simulink model "SYHW_Zscan"  (Simulink 8.1)
settings: Solver=ode5  SolverMode=SingleTasking  StartTime=0.0  StopTime=inf  FixedStep=Ts  RelTol=1e-3
PreLoadFcn:
  | Ts=20e-6;Ts_eHS=8e-7;parameters3;
PostLoadFcn:
  | Ts=20e-6;Ts_eHS=8e-7;parameters3;
InitFcn:
  | Ts=20e-6;Ts_eHS=8e-7;parameters3;
StartFcn:
  | Ts=20e-6;Ts_eHS=8e-7;parameters3;
undefined symbols (not defined in the file or in its folder): Fnom, opsimget, p, SW01
undefined symbols (not defined in the file): LmSI, LrSI, LsSI, RrSI, RsSI
libraries: rtlab x35, rtio_opalrt_common x13, efs_cpuhilios_crtl_lib x4, cpuhilios_lib x4, simulink x3, dspsigops x3, powerlib_extras x1, powerlib_meascontrol x1, rteventslib x1, cpuconverter_lib x1
(part 2 of 2)

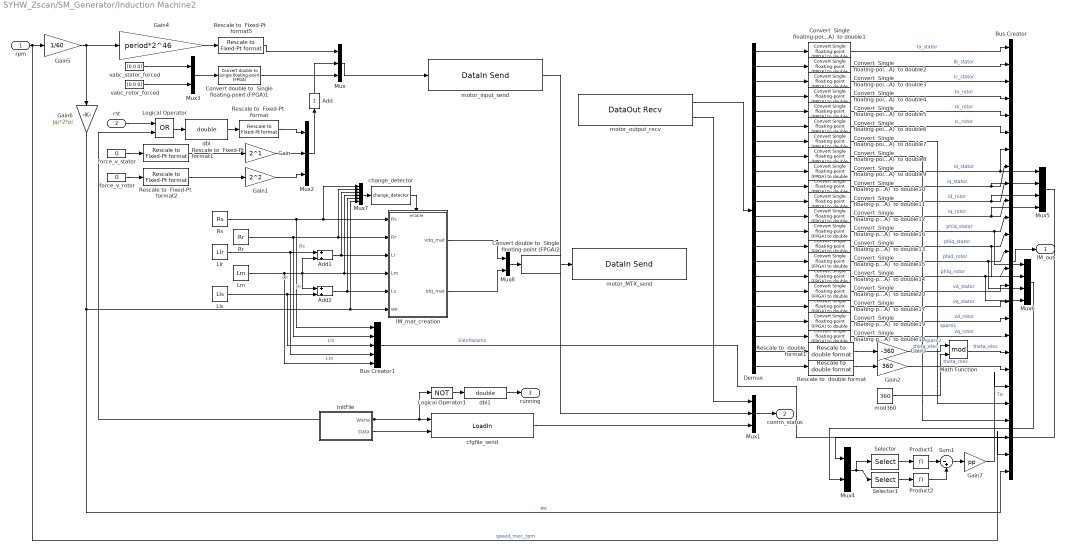
== system SYHW_Zscan/SM_Generator/Induction Machine2 ==
  rpm : Inport  PortDimensions=1
  rst : Inport  Port=2
  Add : Sum  Inputs=+
  Add1 : Sum
  Add2 : Sum
  Bus Creator : BusCreator  Inputs=26
  Bus Creator1 : BusCreator  Inputs=5
  Convert  Single floating-point (FPGA)  to double{1..20} (20 alike) : rtlab/Miscellaneous/Convert  Single floating-point (FPGA)  to double
  Convert double to  Single floating-point (FPGA)1 : rtlab/Miscellaneous/Convert double to  Single floating-point (FPGA)
  Convert double to  Single floating-point (FPGA)2 : rtlab/Miscellaneous/Convert double to  Single floating-point (FPGA)
  Demux : Demux  Outputs=22
  Gain : Gain  Gain=2^1  OutDataTypeStr=uint32
  Gain1 : Gain  Gain=2^2  OutDataTypeStr=uint32
  Gain2 : Gain  Gain=360
  Gain3 : Gain  Gain=-360
  Gain4 : Gain  Gain=period*2^46
  Gain5 : Gain  Gain=1/60
  Gain6 : Gain  Gain=pp*2*pi
  Gain7 : Gain  Gain=pp
  IM_mat_creation : Subsystem
  InitFile : Subsystem
      mask Display:
      | patch([0 0.5 0.7 0],[1 1 0 0],[0.7 0.75 0.9]);
      | patch([1 0.53 0.73 1],[1 1 0 0],[1 0.8 0.7]);
      | port_label('output',2,'Data');
      | 
      | port_label('output',1,'En');
  Llr : Constant  Value=Llr
  Lls : Constant  Value=Lls
  Lm : Constant  Value=Lm
  Logical Operator : Logic  Operator=OR  AllPortsSameDT=off  OutDataTypeStr=boolean
  Logical Operator1 : Logic  Operator=NOT  AllPortsSameDT=off  OutDataTypeStr=boolean
  Math Function : Math  Operator=mod  SaturateOnIntegerOverflow=on
  Mux : Mux  Inputs=3
  Mux1 : Mux  Inputs=3
  Mux2 : Mux  Inputs=3
  Mux3 : Mux  Inputs=2
  Mux4 : Mux  Inputs=2
  Mux5 : Mux
  Mux6 : Mux
  Mux7 : Mux  Inputs=6
  Mux8 : Mux  Inputs=2
  Product1 : Product  Inputs=1  SaturateOnIntegerOverflow=on  InputSameDT=on  OutDataTypeStr=Inherit: Same as first input
  Product2 : Product  Inputs=1  SaturateOnIntegerOverflow=on  InputSameDT=on  OutDataTypeStr=Inherit: Same as first input
  Rescale to  Fixed-Pt  format : rtlab/Miscellaneous/Rescale to  Fixed-Pt  format  FormatType=Unsigned  N=1  Q=0
  Rescale to  Fixed-Pt  format1 : rtlab/Miscellaneous/Rescale to  Fixed-Pt  format  FormatType=Unsigned  N=6  Q=0
  Rescale to  Fixed-Pt  format2 : rtlab/Miscellaneous/Rescale to  Fixed-Pt  format  FormatType=Unsigned  N=1  Q=0
  Rescale to  Fixed-Pt  format5 : rtlab/Miscellaneous/Rescale to  Fixed-Pt  format  FormatType=Signed (2's complement)  N=32  Q=0
  Rescale to  double format : rtlab/Miscellaneous/Rescale to  double format  FormatType=Unsigned  N=32  Q=32
  Rescale to  double format1 : rtlab/Miscellaneous/Rescale to  double format  FormatType=Unsigned  N=32  Q=32
  Rr : Constant  Value=Rr
  Rs : Constant  Value=Rs
  Selector : Selector  InputPortWidth=8  IndexOptions=Index vector (dialog)  Indices=[1 6]  OutputSizes=1
  Selector1 : Selector  InputPortWidth=8  IndexOptions=Index vector (dialog)  Indices=[2 5]  OutputSizes=1
  Sum1 : Sum  Inputs=|-+  SaturateOnIntegerOverflow=on  InputSameDT=on  OutDataTypeStr=Inherit: Same as first input
  cfgfile_send : rtio_opalrt_common/LoadIn  CtrlName='eHS Ctrl'  FcnNos=27  width=10  portType=uint32
      settings: AttributesFormatString=%<CtrlName>
  change_detector : cpuhilios_lib/Aout_Mapping&Adjustments/change_detector
  dbl : DataTypeConversion  OutDataTypeStr=double
  dbl1 : DataTypeConversion  OutDataTypeStr=double
  force_v_rotor : Constant  Value=0
  force_v_stator : Constant  Value=0
  mod360 : Constant  Value=360
  motor_MTX_send : rtio_opalrt_common/DataIn Send  CtrlName='eHS Ctrl'  FcnNos=23  width=32  portType=uint32  checkVersion=off  expectedId=0  expectedVersion=0  opComp=>=
      settings: AttributesFormatString=%<CtrlName>
  motor_input_send : rtio_opalrt_common/DataIn Send  CtrlName='eHS Ctrl'  FcnNos=22  width=8  portType=uint32  checkVersion=off  expectedId=0  expectedVersion=0  opComp=>=
      settings: AttributesFormatString=%<CtrlName>
  motor_output_recv : rtio_opalrt_common/DataOut Recv  CtrlName='eHS Ctrl'  FcnNos=3  width=22  portType=uint32  sampleTime=0  checkVersion=off  expectedId=0  expectedVersion=0  opComp=>=
      settings: AttributesFormatString=%<CtrlName>
  vabc_rotor_forced : Constant  Value=[0 0 0]
  vabc_stator_forced : Constant  Value=[0 0 0]
  IM_out : Outport
  comm_status : Outport  Port=2
  running : Outport  Port=3
  wires:
  Bus Creator1/1 -> Bus Creator/24  "ElecParams"
  Gain5/1 -> Gain4/1, Gain6/1
  dbl1/1 -> running/1
  Logical Operator1/1 -> dbl1/1
  dbl/1 -> Rescale to  Fixed-Pt  format/1
  Rescale to  Fixed-Pt  format/1 -> Mux2/1
  Logical Operator/1 -> dbl/1
  Demux/1 -> Convert  Single floating-point (FPGA)  to double1/1
  rpm/1 -> Bus Creator/25, Gain5/1  "speed_mec_rpm"
  Gain1/1 -> Mux2/3
  Rescale to  Fixed-Pt  format2/1 -> Gain1/1
  force_v_rotor/1 -> Rescale to  Fixed-Pt  format2/1
  Gain/1 -> Mux2/2
  force_v_stator/1 -> Rescale to  Fixed-Pt  format1/1
  Mux2/1 -> Add/1
  Rescale to  Fixed-Pt  format1/1 -> Gain/1
  rst/1 -> Logical Operator/1
  motor_output_recv/1 -> Demux/1
  InitFile/1(Wena) -> Logical Operator1/1, cfgfile_send/1, Logical Operator/2
  Mux/1 -> motor_input_send/1
  Gain4/1 -> Rescale to  Fixed-Pt  format5/1
  Convert double to  Single floating-point (FPGA)1/1 -> Mux/3
  motor_input_send/1 -> Mux1/2
  motor_output_recv/2 -> Mux1/1
  vabc_stator_forced/1 -> Mux3/1
  cfgfile_send/1 -> Mux1/3
  Mux1/1 -> comm_status/1
  InitFile/2(Data) -> cfgfile_send/2
  Rescale to  Fixed-Pt  format5/1 -> Mux/1
  Add/1 -> Mux/2
  Convert  Single floating-point (FPGA)  to double1/1 -> Bus Creator/1  "Ia_stator"
  Rescale to  double format/1 -> Gain2/1
  Rescale to  double format1/1 -> Gain3/1
  Gain2/1 -> Bus Creator/20  "theta_mec"
  Gain3/1 -> Math Function/1  "theta_elec"
  Mux3/1 -> Convert double to  Single floating-point (FPGA)1/1
  vabc_rotor_forced/1 -> Mux3/2
  Convert  Single floating-point (FPGA)  to double2/1 -> Bus Creator/2  "Ib_stator"
  Demux/2 -> Convert  Single floating-point (FPGA)  to double2/1
  Demux/3 -> Convert  Single floating-point (FPGA)  to double3/1
  Convert  Single floating-point (FPGA)  to double3/1 -> Bus Creator/3  "Ic_stator"
  Convert  Single floating-point (FPGA)  to double4/1 -> Bus Creator/4  "Ia_rotor"
  Demux/4 -> Convert  Single floating-point (FPGA)  to double4/1
  Convert  Single floating-point (FPGA)  to double5/1 -> Bus Creator/5  "Ib_rotor"
  Demux/5 -> Convert  Single floating-point (FPGA)  to double5/1
  Convert  Single floating-point (FPGA)  to double6/1 -> Bus Creator/6  "Ic_rotor"
  Demux/6 -> Convert  Single floating-point (FPGA)  to double6/1
  Convert  Single floating-point (FPGA)  to double7/1 -> Bus Creator/22  "spare1"
  Demux/7 -> Convert  Single floating-point (FPGA)  to double7/1
  Convert  Single floating-point (FPGA)  to double8/1 -> Bus Creator/23  "spare2"
  Demux/8 -> Convert  Single floating-point (FPGA)  to double8/1
  Convert  Single floating-point (FPGA)  to double9/1 -> Bus Creator/7, Mux5/1  "id_stator"
  Demux/9 -> Convert  Single floating-point (FPGA)  to double9/1
  Convert  Single floating-point (FPGA)  to double10/1 -> Bus Creator/8, Mux5/2  "iq_stator"
  Demux/10 -> Convert  Single floating-point (FPGA)  to double10/1
  Convert  Single floating-point (FPGA)  to double11/1 -> Bus Creator/9, Mux5/3  "id_rotor"
  Demux/11 -> Convert  Single floating-point (FPGA)  to double11/1
  Convert  Single floating-point (FPGA)  to double12/1 -> Bus Creator/10, Mux5/4  "iq_rotor"
  Demux/12 -> Convert  Single floating-point (FPGA)  to double12/1
  Convert  Single floating-point (FPGA)  to double16/1 -> Bus Creator/11, Mux6/1  "phid_stator"
  Demux/13 -> Convert  Single floating-point (FPGA)  to double16/1
  Convert  Single floating-point (FPGA)  to double13/1 -> Bus Creator/12, Mux6/2  "phiq_stator"
  Demux/14 -> Convert  Single floating-point (FPGA)  to double13/1
  Convert  Single floating-point (FPGA)  to double15/1 -> Bus Creator/13, Mux6/3  "phid_rotor"
  Demux/15 -> Convert  Single floating-point (FPGA)  to double15/1
  Convert  Single floating-point (FPGA)  to double14/1 -> Bus Creator/14, Mux6/4  "phiq_rotor"
  Demux/16 -> Convert  Single floating-point (FPGA)  to double14/1
  Convert  Single floating-point (FPGA)  to double20/1 -> Bus Creator/15  "vd_stator"
  Convert  Single floating-point (FPGA)  to double17/1 -> Bus Creator/16  "vq_stator"
  Convert  Single floating-point (FPGA)  to double19/1 -> Bus Creator/17  "vd_rotor"
  Convert  Single floating-point (FPGA)  to double18/1 -> Bus Creator/18  "vq_rotor"
  Demux/17 -> Convert  Single floating-point (FPGA)  to double20/1
  Demux/18 -> Convert  Single floating-point (FPGA)  to double17/1
  Demux/19 -> Convert  Single floating-point (FPGA)  to double19/1
  Demux/20 -> Convert  Single floating-point (FPGA)  to double18/1
  Demux/21 -> Rescale to  double format1/1
  Demux/22 -> Rescale to  double format/1
  Bus Creator/1 -> IM_out/1
  Mux8/1 -> Convert double to  Single floating-point (FPGA)2/1
  Rs/1 -> Bus Creator1/1, IM_mat_creation/1(Rs), Mux7/1  "Rs"
  Rr/1 -> Bus Creator1/2, IM_mat_creation/2(Rr), Mux7/2  "Rr"
  Llr/1 -> Bus Creator1/4, Add1/1  "Llr"
  Lm/1 -> Bus Creator1/5, IM_mat_creation/4(Lm), Mux7/4, Add2/1, Add1/2  "Lm"
  Lls/1 -> Bus Creator1/3, Add2/2  "Lls"
  IM_mat_creation/1(vdq_mat) -> Mux8/1
  IM_mat_creation/2(idq_mat) -> Mux8/2
  Gain6/1 -> Bus Creator/26, IM_mat_creation/6(we), Mux7/6  "we"
  Selector/1 -> Product1/1
  Selector1/1 -> Product2/1
  Product2/1 -> Sum1/2
  Product1/1 -> Sum1/1
  Sum1/1 -> Gain7/1
  Mux4/1 -> Selector1/1, Selector/1
  Gain7/1 -> Bus Creator/21  "Te"
  Mux5/1 -> Mux4/1
  Mux6/1 -> Mux4/2
  Add1/1 -> IM_mat_creation/3(Lr), Mux7/3
  Add2/1 -> IM_mat_creation/5(Ls), Mux7/5
  Convert double to  Single floating-point (FPGA)2/1 -> motor_MTX_send/1
  Mux7/1 -> change_detector/1
  change_detector/1 -> IM_mat_creation/Enable
  Math Function/1 -> Bus Creator/19  "theta_elec"
  mod360/1 -> Math Function/2

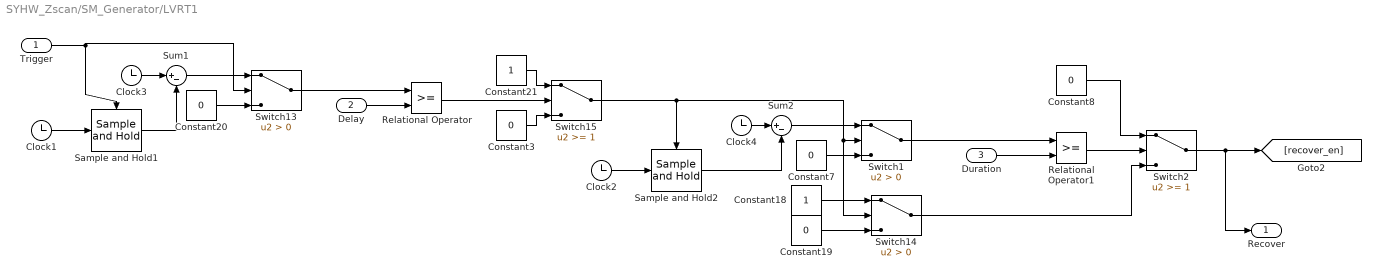
== system SYHW_Zscan/SM_Generator/LVRT1 ==
  Trigger : Inport
  Delay : Inport  Port=2
  Duration : Inport  Port=3
  Clock{1..4} (4 alike) : Clock
      Clock3 settings: DisableCoverage=on
      Clock4 settings: DisableCoverage=on
  Constant18 : Constant
  Constant{3,7..8,19..20} (5 alike) : Constant  Value=0
  Constant21 : Constant
  Relational Operator : RelationalOperator  OutDataTypeStr=boolean
  Relational Operator1 : RelationalOperator  OutDataTypeStr=boolean
  Sample and Hold1 : dspsigops/Sample and Hold  trig=Rising edge  initCond=0  latchinput=off
  Sample and Hold2 : dspsigops/Sample and Hold  trig=Rising edge  initCond=0  latchinput=off
  Sum1 : Sum  DisableCoverage=on  Inputs=|+-  SaturateOnIntegerOverflow=on  InputSameDT=on  OutDataTypeStr=Inherit: Same as first input
  Sum2 : Sum  DisableCoverage=on  Inputs=|+-  SaturateOnIntegerOverflow=on  InputSameDT=on  OutDataTypeStr=Inherit: Same as first input
  Switch1 : Switch  Criteria=u2 > Threshold
  Switch13 : Switch  Criteria=u2 > Threshold
  Switch14 : Switch  Criteria=u2 > Threshold
  Switch15 : Switch  Threshold=1
  Switch2 : Switch  Threshold=1
  Recover : Outport
  wires:
  Duration/1 -> Relational Operator1/2
  Switch1/1 -> Relational Operator1/1
  Relational Operator1/1 -> Switch2/2
  Relational Operator/1 -> Switch15/2
  Delay/1 -> Relational Operator/2
  Switch13/1 -> Relational Operator/1
  Clock2/1 -> Sample and Hold2/1
  Sum2/1 -> Switch1/1
  Constant18/1 -> Switch14/1
  Sample and Hold2/1 -> Sum2/2
  Constant8/1 -> Switch2/1
  Clock4/1 -> Sum2/1
  Constant7/1 -> Switch1/3
  Switch14/1 -> Switch2/3
  Constant19/1 -> Switch14/3
  Sample and Hold1/1 -> Sum1/2
  Clock1/1 -> Sample and Hold1/1
  Constant20/1 -> Switch13/3
  Sum1/1 -> Switch13/1
  Constant21/1 -> Switch15/1
  Constant3/1 -> Switch15/3
  Clock3/1 -> Sum1/1
  Switch15/1 -> Sample and Hold2/Trigger, Switch14/2, Switch1/2
  Trigger/1 -> Switch13/2, Sample and Hold1/Trigger
  Switch2/1 -> Recover/1, [recover_en]

== system SYHW_Zscan/SM_Generator/Motor voltage ==
  Uscan_abc : Inport
  Ugrid_abc : Inport  Port=2
  Add4 : Sum
  Add8 : Sum
  Add9 : Sum
  Bus Creator : BusCreator  Inputs=3
  Demux : Demux  Outputs=3
  Demux1 : Demux  Outputs=3
  Gain1 : Gain  Gain=sqrt(2/3)
  Product : Product  RndMeth=Zero
  Uabc : Sin  Frequency=100*pi  Phase=[0 -2/3*pi 2/3*pi]  SampleTime=0
  Out1 : Outport
  wires:
  Ugrid_abc/1 -> Gain1/1
  Uabc/1 -> Product/1
  Gain1/1 -> Product/2
  Add4/1 -> Bus Creator/1  "Ua_total"
  Add9/1 -> Bus Creator/3  "Uc_total"
  Add8/1 -> Bus Creator/2  "Ub_total"
  Product/1 -> Demux/1
  Demux1/3 -> Add9/2
  Demux1/2 -> Add8/2
  Demux1/1 -> Add4/2
  Uscan_abc/1 -> Demux1/1
  Demux/1 -> Add4/1
  Demux/2 -> Add8/1
  Demux/3 -> Add9/1
  Bus Creator/1 -> Out1/1

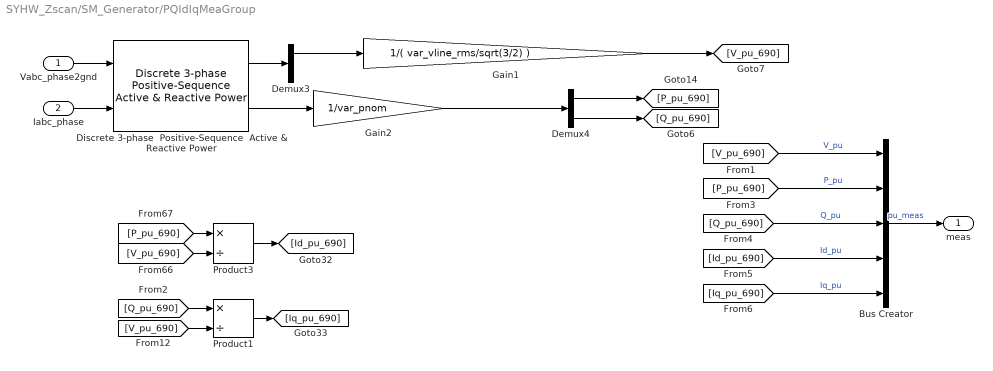
== system SYHW_Zscan/SM_Generator/PQIdIqMeaGroup ==
  Vabc_phase2gnd : Inport
  Iabc_phase : Inport  Port=2
  Bus Creator : BusCreator  Inputs=5
  Demux3 : Demux  Outputs=2
  Demux4 : Demux  Outputs=2
  Discrete 3-phase  Positive-Sequence  Active & Reactive Power : powerlib_extras/Discrete Measurements/Discrete 3-phase  Positive-Sequence  Active & Reactive Power  Freq=50  Par_Vinit=[0 0]  Par_Iinit=[0 0]  Ts=Ts
  Gain1 : Gain  Gain=1/( var_vline_rms/sqrt(3/2) )
  Gain2 : Gain  Gain=1/var_pnom
  Product1 : Product  Inputs=*/  RndMeth=Zero
  Product3 : Product  Inputs=*/  RndMeth=Zero
  meas : Outport
  wires:
  Iabc_phase/1 -> Discrete 3-phase  Positive-Sequence  Active & Reactive Power/2
  Vabc_phase2gnd/1 -> Discrete 3-phase  Positive-Sequence  Active & Reactive Power/1
  Discrete 3-phase  Positive-Sequence  Active & Reactive Power/1 -> Demux3/1
  Demux3/1 -> Gain1/1
  Discrete 3-phase  Positive-Sequence  Active & Reactive Power/2 -> Gain2/1
  Demux4/1 -> [P_pu_690]
  Demux4/2 -> [Q_pu_690]
  Product1/1 -> [Iq_pu_690]
  [Q_pu_690] -> Product1/1
  [V_pu_690] -> Product1/2
  [P_pu_690] -> Product3/1
  Product3/1 -> [Id_pu_690]
  [V_pu_690] -> Product3/2
  [P_pu_690] -> Bus Creator/2  "P_pu"
  [V_pu_690] -> Bus Creator/1  "V_pu"
  [Q_pu_690] -> Bus Creator/3  "Q_pu"
  [Iq_pu_690] -> Bus Creator/5  "Iq_pu"
  [Id_pu_690] -> Bus Creator/4  "Id_pu"
  Bus Creator/1 -> meas/1  "pu_meas"
  Gain1/1 -> [V_pu_690]
  Gain2/1 -> Demux4/1

== system SYHW_Zscan/SM_Generator/QuadEncoders ==
  Slot1B_1 : Inport
  Power base for the Generator3 : Gain  Gain=60*Fnom/p  SaturateOnIntegerOverflow=on  OutDataTypeStr=Inherit: Same as input  ParamDataTypeStr=Inherit: Same as input
  Scope : Scope
      settings: SaveName=ScopeData7
  Speed scaling : Subsystem
  To_FPGA : Outport
  wires:
  Slot1B_1/1 -> Power base for the Generator3/1
  Speed scaling/1(DataIN) -> To_FPGA/1
  Power base for the Generator3/1 -> Scope/1, Speed scaling/2(QuadEnc2), Speed scaling/1(QuadEnc1)

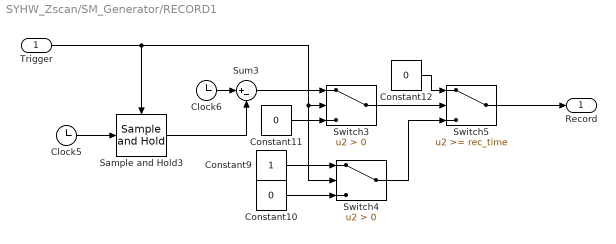
== system SYHW_Zscan/SM_Generator/RECORD1 ==
  Trigger : Inport
  Clock5 : Clock
  Clock6 : Clock
      settings: DisableCoverage=on
  Constant10 : Constant  Value=0
  Constant11 : Constant  Value=0
  Constant12 : Constant  Value=0
  Constant9 : Constant
  Sample and Hold3 : dspsigops/Sample and Hold  trig=Rising edge  initCond=0  latchinput=off
  Sum3 : Sum  DisableCoverage=on  Inputs=|+-  SaturateOnIntegerOverflow=on  InputSameDT=on  OutDataTypeStr=Inherit: Same as first input
  Switch3 : Switch  Criteria=u2 > Threshold
  Switch4 : Switch  Criteria=u2 > Threshold
  Switch5 : Switch  Threshold=rec_time
  Record : Outport
  wires:
  Constant10/1 -> Switch4/3
  Constant12/1 -> Switch5/1
  Sample and Hold3/1 -> Sum3/2
  Clock6/1 -> Sum3/1
  Switch4/1 -> Switch5/3
  Constant11/1 -> Switch3/3
  Constant9/1 -> Switch4/1
  Sum3/1 -> Switch3/1
  Clock5/1 -> Sample and Hold3/1
  Switch3/1 -> Switch5/2
  Trigger/1 -> Switch4/2, Switch3/2, Sample and Hold3/Trigger
  Switch5/1 -> Record/1

== system SYHW_Zscan/SM_Generator/pp2pg ==
  Vabc_pp : Inport
  Add : Sum  Inputs=+-
  Add1 : Sum  Inputs=-+
  Add2 : Sum  Inputs=-+
  Demux : Demux  Outputs=3
  Gain2 : Gain  Gain=1/3
  Mux12 : Mux  Inputs=3
  Vabc : Outport
  wires:
  Mux12/1 -> Gain2/1
  Demux/1 -> Add/1, Add1/1
  Demux/3 -> Add/2, Add2/2
  Add/1 -> Mux12/1
  Gain2/1 -> Vabc/1
  Demux/2 -> Add1/2, Add2/1
  Add1/1 -> Mux12/2
  Add2/1 -> Mux12/3
  Vabc_pp/1 -> Demux/1

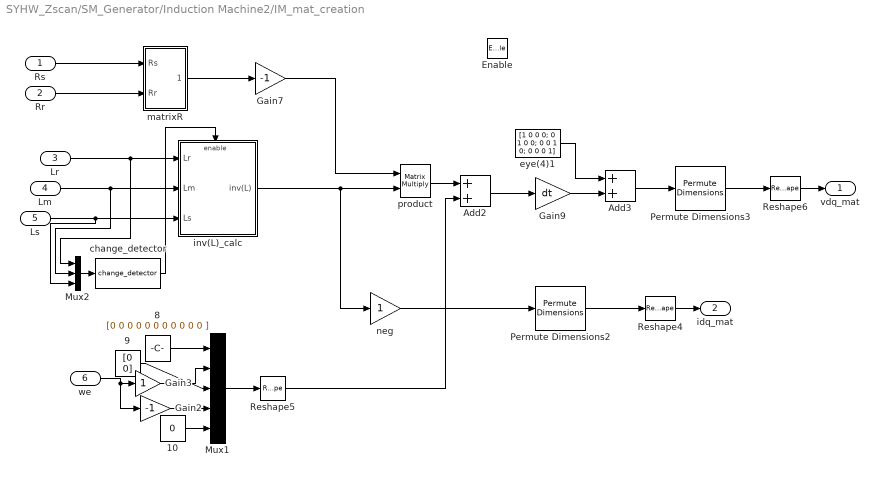
== system SYHW_Zscan/SM_Generator/Induction Machine2/IM_mat_creation ==
  Rs : Inport
  Rr : Inport  Port=2
  Lr : Inport  Port=3
  Lm : Inport  Port=4
  Ls : Inport  Port=5
  we : Inport  Port=6
  Enable : EnablePort
  10 : Constant  Value=0
  8 : Constant  Value=[0 0 0 0 0 0 0 0 0 0 0 ]
  9 : Constant  Value=[0 0]
  Add2 : Sum
  Add3 : Sum
  Gain2 : Gain  Gain=-1
  Gain3 : Gain
  Gain7 : Gain  Gain=-1
  Gain9 : Gain  Gain=dt
  Mux1 : Mux  Inputs=[11 1 2 1 1]
  Mux2 : Mux  Inputs=3
  Permute Dimensions2 : PermuteDimensions
  Permute Dimensions3 : PermuteDimensions
  Reshape4 : Reshape
  Reshape5 : Reshape  OutputDimensionality=Customize  OutputDimensions=[4,4]
  Reshape6 : Reshape
  change_detector : cpuhilios_lib/Aout_Mapping&Adjustments/change_detector
  eye(4)1 : Constant  Value="[1 0 0 0; 0 1 0 0; 0 0  1  0;  0  0  0  1]"
  inv(L)_calc : Subsystem
  matrixR : Subsystem
  neg : Gain
  product : Product  Multiplication=Matrix(*)
  vdq_mat : Outport
  idq_mat : Outport  Port=2
  wires:
  Gain3/1 -> Mux1/2
  10/1 -> Mux1/5
  9/1 -> Mux1/3
  Gain2/1 -> Mux1/4
  we/1 -> Gain2/1, Gain3/1
  8/1 -> Mux1/1
  Mux1/1 -> Reshape5/1
  inv(L)_calc/1(inv(L)) -> product/2, neg/1
  product/1 -> Add2/1
  matrixR/1(mat) -> Gain7/1
  Reshape5/1 -> Add2/2
  Add2/1 -> Gain9/1
  Gain9/1 -> Add3/2
  eye(4)1/1 -> Add3/1
  Gain7/1 -> product/1
  Permute Dimensions2/1 -> Reshape4/1
  Permute Dimensions3/1 -> Reshape6/1
  Add3/1 -> Permute Dimensions3/1
  Rs/1 -> matrixR/1(Rs)
  Rr/1 -> matrixR/2(Rr)
  Reshape6/1 -> vdq_mat/1
  Reshape4/1 -> idq_mat/1
  Lr/1 -> inv(L)_calc/1(Lr), Mux2/1
  Lm/1 -> inv(L)_calc/2(Lm), Mux2/2
  Ls/1 -> inv(L)_calc/3(Ls), Mux2/3
  change_detector/1 -> inv(L)_calc/Enable
  Mux2/1 -> change_detector/1
  neg/1 -> Permute Dimensions2/1

== system SYHW_Zscan/SM_Generator/Induction Machine2/InitFile ==
  note: Write Enable while the index
      | is different from the file
      | length + one cycle for the
      | final sample
  Constant1 : Constant  Value=0
  Constant2 : Constant
  Data Type Conversion : DataTypeConversion  OutDataTypeStr=uint32
  Data Type Conversion1 : DataTypeConversion  OutDataTypeStr=double
  Memory : Memory  X0=1
  Memory1 : Memory  X0=1
  MotorInitFile : rtlab/DataLogging/OpFromFile  filename_mode=Static (same filename all the time)  reload_mode=Next time model is paused (Real-Time)  init_file_id=0  filename=IM_cfg12550.mat  rtpath='./'  nrtpath='EFPGASIMConfig\'  sample_time=opsimget(bdroot)
  Relational Operator : RelationalOperator  Operator=~=  OutDataTypeStr=boolean
  Terminator : Terminator
  Wena : Outport
  Data : Outport  Port=2
  wires:
  Memory1/1 -> MotorInitFile/4
  Memory/1 -> Data Type Conversion1/1
  MotorInitFile/3 -> Memory1/1, Relational Operator/2
  Relational Operator/1 -> Memory/1
  MotorInitFile/4 -> Relational Operator/1
  MotorInitFile/2 -> Data Type Conversion/1
  Constant1/1 -> MotorInitFile/6, MotorInitFile/2, MotorInitFile/3
  MotorInitFile/1 -> Terminator/1
  Constant2/1 -> MotorInitFile/5, MotorInitFile/1
  Data Type Conversion/1 -> Data/1
  Data Type Conversion1/1 -> Wena/1

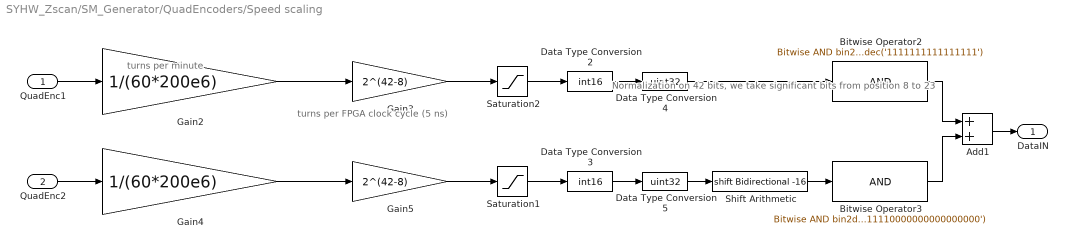
== system SYHW_Zscan/SM_Generator/QuadEncoders/Speed scaling ==
  note: Normalization on 42 bits,
      | we take significant bits from
      | position 8 to 23
  note: turns per FPGA
      | clock cycle (5 ns)
  note: turns per minute
  QuadEnc1 : Inport
  QuadEnc2 : Inport  Port=2
  Add1 : Sum
  Bitwise Operator2 : simulink/Logic and Bit Operations/Bitwise Operator  logicop=AND  UseBitMask=on  BitMask=bin2dec('1111111111111111')  BitMaskRealWorld=Stored Integer
  Bitwise Operator3 : simulink/Logic and Bit Operations/Bitwise Operator  logicop=AND  UseBitMask=on  BitMask=bin2dec('11111111111111110000000000000000')  BitMaskRealWorld=Stored Integer
  Data Type Conversion2 : DataTypeConversion  OutDataTypeStr=int16
  Data Type Conversion3 : DataTypeConversion  OutDataTypeStr=int16
  Data Type Conversion4 : DataTypeConversion  OutDataTypeStr=uint32
  Data Type Conversion5 : DataTypeConversion  OutDataTypeStr=uint32
  Gain2 : Gain  Gain=1/(60*200e6)
  Gain3 : Gain  Gain=2^(42-8)
  Gain4 : Gain  Gain=1/(60*200e6)
  Gain5 : Gain  Gain=2^(42-8)
  Saturation1 : Saturate  UpperLimit=2^15-1  LowerLimit=-2^15
  Saturation2 : Saturate  UpperLimit=2^15-1  LowerLimit=-2^15
  Shift Arithmetic : ArithShift  BitShiftNumber=-16
  DataIN : Outport
  wires:
  Add1/1 -> DataIN/1
  Saturation1/1 -> Data Type Conversion3/1
  Saturation2/1 -> Data Type Conversion2/1
  QuadEnc1/1 -> Gain2/1
  QuadEnc2/1 -> Gain4/1
  Data Type Conversion2/1 -> Data Type Conversion4/1
  Bitwise Operator3/1 -> Add1/2
  Bitwise Operator2/1 -> Add1/1
  Shift Arithmetic/1 -> Bitwise Operator3/1
  Data Type Conversion5/1 -> Shift Arithmetic/1
  Data Type Conversion3/1 -> Data Type Conversion5/1
  Data Type Conversion4/1 -> Bitwise Operator2/1
  Gain5/1 -> Saturation1/1
  Gain4/1 -> Gain5/1
  Gain3/1 -> Saturation2/1
  Gain2/1 -> Gain3/1

== system SYHW_Zscan/SM_Generator/Induction Machine2/IM_mat_creation/inv(L)_calc ==
  Lr : Inport
  Lm : Inport  Port=2
  Ls : Inport  Port=3
  Enable : EnablePort
  det : Subsystem
  inverse : Product  Inputs=/
  matrixL : Subsystem
  mult : Product
  inv(L) : Outport
  wires:
  Lm/1 -> det/3(lm), matrixL/2(Lm)
  Lr/1 -> det/1(lr), matrixL/1(Lr)
  Ls/1 -> det/2(ls), matrixL/3(Ls)
  matrixL/1(mat) -> mult/1
  det/1(lr*ls + lm*lm) -> inverse/1
  inverse/1 -> mult/2
  mult/1 -> inv(L)/1

== system SYHW_Zscan/SM_Generator/Induction Machine2/IM_mat_creation/matrixR ==
  Rs : Inport
  Rr : Inport  Port=2
  11 : Constant  Value=[0 0 0 0]
  Mux2 : Mux  Inputs=[1 4 1 4 1 4 1]
  Reshape4 : Reshape  OutputDimensionality=Customize  OutputDimensions=[4,4]
  mat : Outport
  wires:
  Rs/1 -> Mux2/3, Mux2/1
  Rr/1 -> Mux2/7, Mux2/5
  11/1 -> Mux2/2, Mux2/6, Mux2/4
  Mux2/1 -> Reshape4/1
  Reshape4/1 -> mat/1

== system SYHW_Zscan/SM_Generator/Induction Machine2/IM_mat_creation/inv(L)_calc/det ==
  lr : Inport
  ls : Inport  Port=2
  lm : Inport  Port=3
  Add2 : Sum  Inputs=+-
  mult : Product
  mult1 : Product
  lr*ls + lm*lm : Outport
  wires:
  lm/1 -> mult1/2, mult1/1
  mult/1 -> Add2/1
  mult1/1 -> Add2/2
  lr/1 -> mult/1
  ls/1 -> mult/2
  Add2/1 -> lr*ls + lm*lm/1

== system SYHW_Zscan/SM_Generator/Induction Machine2/IM_mat_creation/inv(L)_calc/matrixL ==
  Lr : Inport
  Lm : Inport  Port=2
  Ls : Inport  Port=3
  11 : Constant  Value=0
  Mux2 : Mux  Inputs=16
  Reshape4 : Reshape  OutputDimensionality=Customize  OutputDimensions=[4,4]
  Unary Minus : UnaryMinus
  mat : Outport
  wires:
  Lr/1 -> Mux2/6, Mux2/1
  11/1 -> Mux2/2, Mux2/4, Mux2/5, Mux2/7, Mux2/10, Mux2/12, Mux2/13, Mux2/15
  Unary Minus/1 -> Mux2/3, Mux2/8, Mux2/9, Mux2/14  "-lm"
  Ls/1 -> Mux2/16, Mux2/11
  Mux2/1 -> Reshape4/1
  Lm/1 -> Unary Minus/1
  Reshape4/1 -> mat/1

== matlab function SM_Generator/Disturb1/MATLAB Function1 ==
  data: t input double; Ua output double; fcn_i data_store_memory double; Ub output double; flag1 data_store_memory double; Uc output double; U_scan data_store_memory double; f_scan data_store_memory double; close input double; nn data_store_memory double; s_fcn_i output double; s_fscan output double; s_nn output double; flag2 data_store_memory double; Num input double; UofPCC parameter double; ScanRatio1 input double; ScanRatio2 input double; s_HorL output double


function [Ua,Ub,Uc,s_fcn_i,s_fscan,s_nn,s_HorL] = fcnU(t,close,Num,UofPCC,ScanRatio1,ScanRatio2)
%#codegen
global fcn_i;
global flag1;
global flag2;%nnn
global f_scan;
global U_scan;
global nn;

Decimation_l = 5;
f_array_low =1:1:350;
f_array_high =250:10:2510;
f_array =[f_array_low,f_array_high];
f_length=length(f_array);
f = f_array;
Numof1sec=floor(Num)*10000;
Num_add=2*Numof1sec;%扰动持续时间
Num_free=0.2*Numof1sec;%正常持续时间
% 
if fcn_i>length(f_array_low)%判断低频段还是高频段
   HorL =1;
else
   HorL =0;
end

if HorL==0 %判断录波开始时间
    Num_save_begin=1*Numof1sec+Decimation_l;
else
    Num_save_begin=1*Numof1sec;%录波开始时间
end

if close==1
    if fcn_i==f_length%(f_end-f_start)/f_int+1
            nn=0;
            flag1=1;
            flag2=0;
    else
        if flag1==0
            if nn==Num_add
                nn=0;
                flag1=1;
                flag2=0;
                fcn_i=fcn_i+1;
            elseif nn>Num_save_begin
                nn=nn+1;
                flag1=0;
                flag2=flag2+1;
            else
                nn=nn+1;
                flag1=0;
                flag2=0;
            end
        else
            if nn==Num_free
                nn=0;
                flag1=0;
            else
                nn=nn+1;
                flag1=1;
            end
            flag2=0;
        end
    end
    
    if flag1==0
        if fcn_i>0
        f_scan = f(fcn_i) % 外加扰动频率
        end
        if fcn_i < 20
            U_scan = UofPCC/sqrt(3)*sqrt(2)*ScanRatio1; %低频段扰动
        else
            U_scan = UofPCC/sqrt(3)*sqrt(2)*ScanRatio2; %
        end
    else
        f_scan=0; 
        U_scan=0; 
    end    
else
        flag1=0;
        flag2=0;
        fcn_i=1;
        f_scan=0; 
        U_scan=0; 
        nn=0; 
end

    
Ua=U_scan*sin(2*pi*f_scan*t);
Ub=0.5*U_scan*(sin(2*pi*f_scan*t-2*pi/3))+0.5*U_scan*(sin(2*pi*f_scan*t+2*pi/3));
Uc=Ub;

s_fcn_i=fcn_i;
s_fscan=f_scan;
s_nn=flag2;
s_HorL=HorL;
